simulink model "kalmanAndroidAHRS"  (R2019b)
settings: Solver=FixedStepAuto  StartTime=0.0  StopTime=40  RelTol=1e-3
InitFcn:
  | Ts=0.01
undefined symbols (not defined in the file): Accel, AHRS_Ang_Vel, AHRS_Attitude, Alt, AttiudeFiltered, fdesignblkfcn, gcbh, Gyro, Heading_Angle, kalman, kalman_clean, Mag, Pitch_Angle, Pitch_Rate, Roll_Angle, Roll_Rate, Slider, Static_Orientation, Yaw_Rate
libraries: androiduilib x15, simulink_extras x6, androidsensorlib x5, mspfiltlib x1, aerolibatmos2 x1
PreSaveFcn:
  | set_param(gcs, 'Location',[35 56 895 605])
settings Model: SimulationMode=external  ExtModeTrigDuration=100  Creator=The MathWorks, Inc.  LastModifiedBy=alireza
settings DataIOCC: LimitDataPoints=on  SaveFormat=Array  ReturnWorkspaceOutputs=off
settings OptimizationCC: LifeSpan=1  MaxStackSize=64
settings DebuggingCC: UnderspecifiedInitializationDetection=Classic  MergeDetectMultiDrivingBlocksExec=none  ParameterPrecisionLossMsg=none  AllowSymbolicDim=off  SFUnexpectedBacktrackingDiag=warning  SFNoUnconditionalDefaultTransitionDiag=warning  SFExecutionAtInitializationDiag=none  ArithmeticOperatorsInVariantConditions=warning
settings HardwareCC: ProdBitPerPointer=32  ProdBitPerSizeT=32  ProdBitPerPtrDiffT=32  ProdLargestAtomicInteger=Long  ProdLargestAtomicFloat=Double  ProdWordSize=32  ProdHWDeviceType=ARM Compatible->ARM Cortex  TargetLargestAtomicInteger=Long  TargetLargestAtomicFloat=Double  TargetEndianess=LittleEndian  TargetHWDeviceType=ARM Compatible->ARM Cortex
settings ModelReferenceCC: PropagateSignalLabelsOutOfModel=off
settings SFSimCC: SimUseLocalCustomCode=off  CustomCodeUndefinedFunction=UseInterfaceOnly
settings RTWCC: SystemTargetFile=ert.tlc  HardwareBoard=Android Device  TLCOptions="-aInlineSetEventsForThisBaseRateFcn=TLC_FALSE -aSuppressMultiTaskScheduler=TLC_FALSE  -aRateBasedStepFcn=0"  TemplateMakefile=ert_default_tmf  GenerateReport=on  RTWVerbose=off  RTWUseLocalCustomCode=off  Toolchain=Android SDK/NDK Tools  LaunchReport=on
settings CodeAppCC: ForceParamTrailComments=on  OperatorAnnotations=on  MangleLength=10  StateflowObjectComments=on  MATLABSourceComments=on
settings ERTTargetCC: MultiwordLength=2048  ERTCustomFileBanners=off  SupportContinuousTime=on  SupportNonInlinedSFcns=on  RemoveResetFunc=off  SupportVariableSizeSignals=on  ModelStepFunctionPrototypeControlCompliant=off
settings ConfigComp: CovMetricSettings=dw  CovHtmlReporting=on  CovSaveCumulativeToWorkspaceVar=on  CovSaveSingleToWorkspaceVar=on  CovExternalEMLEnable=off  CovSFcnEnable=off

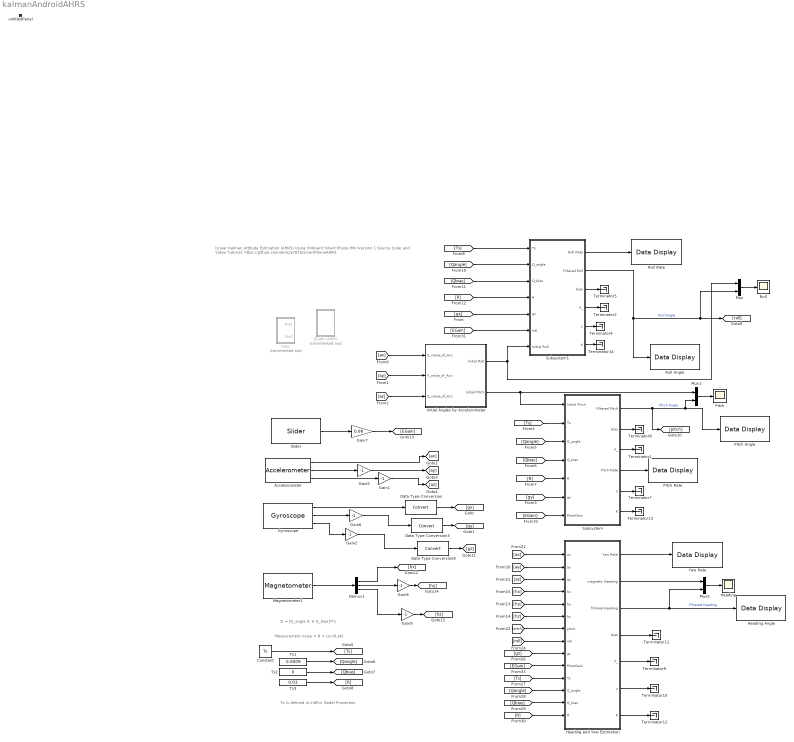
== system kalmanAndroidAHRS ==
  note: Ts is defined in initFcn Model Properties
  note: Linear Kalman Attitude Estimation (AHRS)
      | Using Onboard Smart Phone IMU Version 1
      | Source Code and Video Tutorial:
      | https://github.com/alireza787b/smartPhoneAHRS
  note: Measurement noise = R = cov(0,ek)
  note: Q = [Q_angle 0; 0 Q_bias]*Ts
  Accelerometer : androidsensorlib/Accelerometer  OutputVector=off  SampleTime=Ts  BlockPlatform=Android
      settings: SourceProductBaseCode=ANDROID
  BuiltIn AHRS : Subsystem  Commented=on
  Constant : Constant  Value=Ts
  Data Type Conversion : DataTypeConversion
  Data Type Conversion3 : DataTypeConversion
  Data Type Conversion8 : DataTypeConversion
  Demux1 : Demux  Outputs=3
  Gain{1..2,5..6,8..9} (6 alike) : Gain  Gain=-1
  Gain7 : Gain  Gain=0.98
  Gyroscope : androidsensorlib/Gyroscope  OutputVector=off  SampleTime=Ts  BlockPlatform=Android
      settings: SourceProductBaseCode=ANDROID
  Heading : Scope
  Heading Angle : androiduilib/Data Display  DataDisplayId=kalman_clean/Heading_Angle  Format=Float  Precision=6  SimulateUsing=Code generation  blockPlatform=Android
      settings: SourceProductBaseCode=ANDROID
  Heading and Yaw Estimation : Subsystem
  Initial Angles by Accelerometer : Subsystem
  Magnetometer1 : androidsensorlib/Magnetometer  SampleTime=0.01  SimulateUsing=Code generation
      settings: SourceProductBaseCode=ANDROID
  Mux : Mux  Inputs=2
  Mux1 : Mux  Inputs=2
  Mux5 : Mux  Inputs=2
  Pitch : Scope
  Pitch Angle : androiduilib/Data Display  DataDisplayId=kalman_clean/Pitch_Angle  Format=Float  Precision=6  SimulateUsing=Code generation  blockPlatform=Android
      settings: SourceProductBaseCode=ANDROID
  Pitch Rate : androiduilib/Data Display  DataDisplayId=kalman_clean/Pitch_Rate  Format=Float  Precision=6  SimulateUsing=Code generation  blockPlatform=Android
      settings: SourceProductBaseCode=ANDROID
  Roll : Scope
  Roll Angle : androiduilib/Data Display  DataDisplayId=kalman_clean/Roll_Angle  Format=Float  Precision=6  SimulateUsing=Code generation  blockPlatform=Android
      settings: SourceProductBaseCode=ANDROID
  Roll Rate : androiduilib/Data Display  DataDisplayId=kalman_clean/Roll_Rate  Format=Float  Precision=6  SimulateUsing=Code generation  blockPlatform=Android
      settings: SourceProductBaseCode=ANDROID
  Slider : androiduilib/Slider  Min=0  Value=1  Max=2  Resolution=0.1  SliderId=kalman_clean/Slider  SampleTime=0.1  BlockPlatform=Android
      settings: SourceProductBaseCode=ANDROID
  Subsystem : Subsystem
  Subsystem1 : Subsystem
  Terminator{1..2,4..5,7..14} (12 alike) : Terminator
  Ts1 : Constant  Value=0.0009
  Ts2 : Constant  Value=0
  Ts3 : Constant  Value=0.03
  Yaw Rate : androiduilib/Data Display  DataDisplayId=kalman_clean/Yaw_Rate  Format=Float  Precision=6  SimulateUsing=Code generation  blockPlatform=Android
      settings: SourceProductBaseCode=ANDROID
  misc : Subsystem  Commented=on
  untitledPanel : Subsystem  Tag=HiddenForWebPanel  IsWebBlockPanel=on
  wires:
  Accelerometer/3 -> Gain1/1
  Accelerometer/1 -> [ax]
  Accelerometer/2 -> Gain5/1
  Gyroscope/2 -> Gain6/1
  Gyroscope/3 -> Gain2/1
  Gyroscope/1 -> Data Type Conversion/1
  Data Type Conversion/1 -> [gx]
  Data Type Conversion3/1 -> [gy]
  Gain6/1 -> Data Type Conversion3/1
  Mux/1 -> Roll/1
  Mux1/1 -> Pitch/1
  Constant/1 -> [Ts]
  Ts2/1 -> [Qbias]
  Ts1/1 -> [Qangle]
  Ts3/1 -> [R]
  Magnetometer1/1 -> Demux1/1
  Data Type Conversion8/1 -> [gz]
  Mux5/1 -> Heading/1
  Slider/1 -> Gain7/1
  Gain5/1 -> [ay]
  Demux1/1 -> [hx]
  Demux1/2 -> Gain8/1
  Demux1/3 -> Gain9/1
  Gain8/1 -> [hy]
  Gain1/1 -> [az]
  Gain2/1 -> Data Type Conversion8/1
  Gain9/1 -> [hz]
  Gain7/1 -> [EGain]
  [ax] -> Heading and Yaw Estimation/1(ax)
  [ay] -> Heading and Yaw Estimation/2(ay)
  [az] -> Heading and Yaw Estimation/3(az)
  [hx] -> Heading and Yaw Estimation/4(hx)
  [hy] -> Heading and Yaw Estimation/5(hy)
  [hz] -> Heading and Yaw Estimation/6(hz)
  [pitch] -> Heading and Yaw Estimation/7(pitch)
  [roll] -> Heading and Yaw Estimation/8(roll)
  [gz] -> Heading and Yaw Estimation/9(gz)
  [EGain] -> Heading and Yaw Estimation/10(filterGain)
  [Ts] -> Heading and Yaw Estimation/11(Ts)
  [Qangle] -> Heading and Yaw Estimation/12(Q_angle)
  [Qbias] -> Heading and Yaw Estimation/13(Q_bias)
  [R] -> Heading and Yaw Estimation/14(R)
  Heading and Yaw Estimation/1(Yaw Rate) -> Yaw Rate/1
  Heading and Yaw Estimation/2(magnetic Heading) -> Mux5/1
  Heading and Yaw Estimation/4(bias) -> Terminator11/1
  Heading and Yaw Estimation/5(P_) -> Terminator9/1
  Heading and Yaw Estimation/6(y) -> Terminator10/1
  Heading and Yaw Estimation/7(K) -> Terminator12/1
  Heading and Yaw Estimation/3(filtered Heading) -> Mux5/2, Heading Angle/1  "Filtered Heading"
  Subsystem/1(Filtered Pitch) -> [pitch], Pitch Angle/1, Mux1/2  "Pitch Angle"
  [Ts] -> Subsystem/2(Ts)
  [Qangle] -> Subsystem/3(Q_angle)
  [Qbias] -> Subsystem/4(Q_bias)
  [R] -> Subsystem/5(R)
  [gy] -> Subsystem/6(gy)
  [EGain] -> Subsystem/7(filterGain)
  Subsystem/2(bias) -> Terminator8/1
  Subsystem/3(P_) -> Terminator1/1
  Subsystem/4(Pitch Rate) -> Pitch Rate/1
  Subsystem/5(y) -> Terminator7/1
  Subsystem/6(K) -> Terminator13/1
  Subsystem1/2(Filtered Roll) -> [roll], Mux/2, Roll Angle/1  "Roll Angle"
  Subsystem1/1(Roll Rate) -> Roll Rate/1
  [Ts] -> Subsystem1/1(Ts)
  [Qangle] -> Subsystem1/2(Q_angle)
  [Qbias] -> Subsystem1/3(Q_bias)
  [R] -> Subsystem1/4(R)
  [gx] -> Subsystem1/5(gx)
  [EGain] -> Subsystem1/6(In6)
  Subsystem1/3(bias) -> Terminator5/1
  Subsystem1/4(P_) -> Terminator2/1
  Subsystem1/5(y) -> Terminator4/1
  Subsystem1/6(K) -> Terminator14/1
  Initial Angles by Accelerometer/1(Initial Roll) -> Mux/1, Subsystem1/7(Initial Roll)
  Initial Angles by Accelerometer/2(Initial Pitch) -> Subsystem/1(Initial Pitch), Mux1/1
  [ax] -> Initial Angles by Accelerometer/1(X_value_of_Acc)
  [ay] -> Initial Angles by Accelerometer/2(Y_value_of_Acc)
  [az] -> Initial Angles by Accelerometer/3(Z_value_of_Acc)

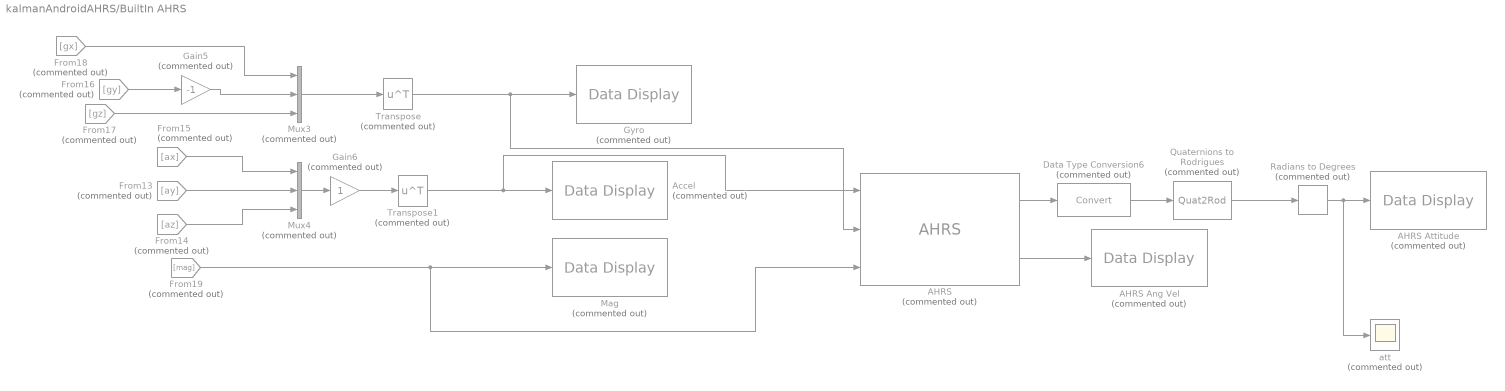
== system kalmanAndroidAHRS/BuiltIn AHRS ==
  AHRS : mspfiltlib/AHRS  Commented=on  DispRefFrame=NED  DecimationFactor=1  InitialProcessNoise=ahrsfilter.defaultProcessNoise  OrientationFormat=quaternion  SimulateUsing=Code generation  AccelerometerNoise=7.7792e-07  GyroscopeNoise=3.7046e-08  MagnetometerNoise=0.1  GyroscopeDriftNoise=3.0462e-13  LinearAccelerationNoise=0.0096236100000000012  MagneticDisturbanceNoise=0.5  LinearAccelerationDecayFactor=0.5  MagneticDisturbanceDecayFactor=0.5  ExpectedMagneticFieldStrength=50
      settings: SourceProductBaseCode=TF,NV
  AHRS Ang Vel : androiduilib/Data Display  Commented=on  DataDisplayId=kalman/AHRS_Ang_Vel  Format=Float  Precision=6  SimulateUsing=Code generation  blockPlatform=Android
      settings: SourceProductBaseCode=ANDROID
  AHRS Attitude : androiduilib/Data Display  Commented=on  DataDisplayId=kalman/AHRS_Attitude  Format=Float  Precision=6  SimulateUsing=Code generation  blockPlatform=Android
      settings: SourceProductBaseCode=ANDROID
  Accel : androiduilib/Data Display  Commented=on  DataDisplayId=kalman/Accel  Format=Float  Precision=6  SimulateUsing=Code generation  blockPlatform=Android
      settings: SourceProductBaseCode=ANDROID
  Data Type Conversion6 : DataTypeConversion  Commented=on
  From13 : From  Commented=on  GotoTag=ay
  From14 : From  Commented=on  GotoTag=az
  From15 : From  Commented=on  GotoTag=ax
  From16 : From  Commented=on  GotoTag=gy
  From17 : From  Commented=on  GotoTag=gz
  From18 : From  Commented=on  GotoTag=gx
  From19 : From  Commented=on  GotoTag=mag
  Gain5 : Gain  Commented=on  Gain=-1
  Gain6 : Gain  Commented=on
  Gyro : androiduilib/Data Display  Commented=on  DataDisplayId=kalman/Gyro  Format=Float  Precision=6  SimulateUsing=Code generation  blockPlatform=Android
      settings: SourceProductBaseCode=ANDROID
  Mag : androiduilib/Data Display  Commented=on  DataDisplayId=kalman/Mag  Format=Float  Precision=6  SimulateUsing=Code generation  blockPlatform=Android
      settings: SourceProductBaseCode=ANDROID
  Mux3 : Mux  Commented=on  Inputs=3
  Mux4 : Mux  Commented=on  Inputs=3
  Quaternions to Rodrigues : Quat2Rod  Commented=on
  Radians to Degrees : simulink_extras/Transformations/Radians to Degrees  Commented=on
  Transpose : Math  Commented=on  Operator=transpose  SaturateOnIntegerOverflow=on
  Transpose1 : Math  Commented=on  Operator=transpose  SaturateOnIntegerOverflow=on
  att : Scope  Commented=on
  wires:
  From18/1 -> Mux3/1
  From14/1 -> Mux4/3
  AHRS/2 -> AHRS Ang Vel/1
  Transpose/1 -> AHRS/2, Gyro/1
  From17/1 -> Mux3/3
  Mux4/1 -> Gain6/1
  Transpose1/1 -> AHRS/1, Accel/1
  From15/1 -> Mux4/1
  From19/1 -> AHRS/3, Mag/1
  From13/1 -> Mux4/2
  AHRS/1 -> Data Type Conversion6/1
  Data Type Conversion6/1 -> Quaternions to Rodrigues/1
  Quaternions to Rodrigues/1 -> Radians to Degrees/1
  Radians to Degrees/1 -> att/1, AHRS Attitude/1
  Gain6/1 -> Transpose1/1
  Gain5/1 -> Mux3/2
  From16/1 -> Gain5/1
  Mux3/1 -> Transpose/1

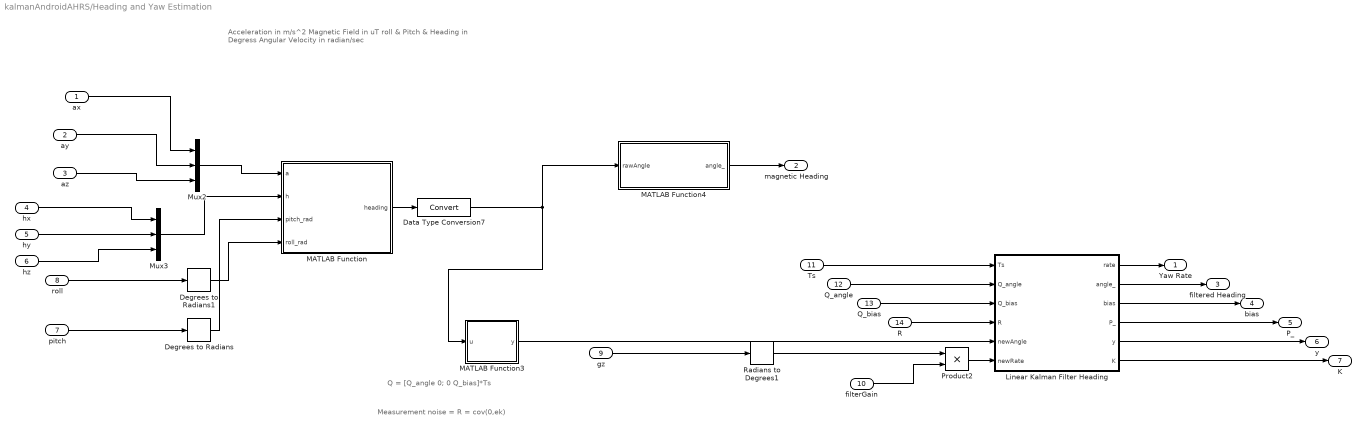
== system kalmanAndroidAHRS/Heading and Yaw Estimation ==
  note: Acceleration in m/s^2
      | Magnetic Field in uT
      | roll & Pitch & Heading in Degress
      | Angular Velocity in radian/sec
  note: Measurement noise = R = cov(0,ek)
  note: Q = [Q_angle 0; 0 Q_bias]*Ts
  ax : Inport
  ay : Inport  Port=2
  az : Inport  Port=3
  hx : Inport  Port=4
  hy : Inport  Port=5
  hz : Inport  Port=6
  pitch : Inport  Port=7
  roll : Inport  Port=8
  gz : Inport  Port=9
  filterGain : Inport  Port=10
  Ts : Inport  Port=11
  Q_angle : Inport  Port=12
  Q_bias : Inport  Port=13
  R : Inport  Port=14
  Data Type Conversion7 : DataTypeConversion
  Degrees to Radians : simulink_extras/Transformations/Degrees to Radians
  Degrees to Radians1 : simulink_extras/Transformations/Degrees to Radians
  Linear Kalman Filter Heading : MATLAB Function  TreatAsAtomicUnit=on
  MATLAB Function : MATLAB Function  TreatAsAtomicUnit=on
  MATLAB Function3 : MATLAB Function  TreatAsAtomicUnit=on
  MATLAB Function4 : MATLAB Function  TreatAsAtomicUnit=on
  Mux2 : Mux  Inputs=3
  Mux3 : Mux  Inputs=3
  Product2 : Product
  Radians to Degrees1 : simulink_extras/Transformations/Radians to Degrees
  Yaw Rate : Outport
  magnetic Heading : Outport  Port=2
  filtered Heading : Outport  Port=3
  bias : Outport  Port=4
  P_ : Outport  Port=5
  y : Outport  Port=6
  K : Outport  Port=7
  wires:
  MATLAB Function3/1(y) -> Linear Kalman Filter Heading/5(newAngle)
  Mux2/1 -> MATLAB Function/1(a)
  hy/1 -> Mux3/2
  Degrees to Radians/1 -> MATLAB Function/3(pitch_rad)
  Data Type Conversion7/1 -> MATLAB Function3/1(u), MATLAB Function4/1(rawAngle)
  Linear Kalman Filter Heading/2(angle_) -> filtered Heading/1
  Product2/1 -> Linear Kalman Filter Heading/6(newRate)
  Linear Kalman Filter Heading/6(K) -> K/1
  MATLAB Function/1(heading) -> Data Type Conversion7/1
  Radians to Degrees1/1 -> Product2/1
  Degrees to Radians1/1 -> MATLAB Function/4(roll_rad)
  Mux3/1 -> MATLAB Function/2(h)
  MATLAB Function4/1(angle_) -> magnetic Heading/1
  ay/1 -> Mux2/2
  ax/1 -> Mux2/1
  Q_angle/1 -> Linear Kalman Filter Heading/2(Q_angle)
  gz/1 -> Radians to Degrees1/1
  Ts/1 -> Linear Kalman Filter Heading/1(Ts)
  az/1 -> Mux2/3
  R/1 -> Linear Kalman Filter Heading/4(R)
  Linear Kalman Filter Heading/3(bias) -> bias/1
  Linear Kalman Filter Heading/1(rate) -> Yaw Rate/1
  hz/1 -> Mux3/3
  hx/1 -> Mux3/1
  filterGain/1 -> Product2/2
  Q_bias/1 -> Linear Kalman Filter Heading/3(Q_bias)
  roll/1 -> Degrees to Radians1/1
  pitch/1 -> Degrees to Radians/1
  Linear Kalman Filter Heading/5(y) -> y/1
  Linear Kalman Filter Heading/4(P_) -> P_/1

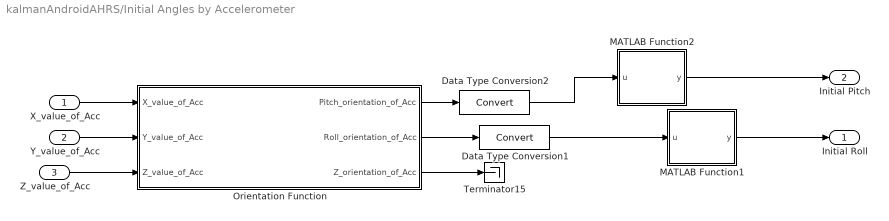
== system kalmanAndroidAHRS/Initial Angles by Accelerometer ==
  X_value_of_Acc : Inport
  Y_value_of_Acc : Inport  Port=2
  Z_value_of_Acc : Inport  Port=3
  Data Type Conversion1 : DataTypeConversion
  Data Type Conversion2 : DataTypeConversion
  MATLAB Function1 : MATLAB Function  TreatAsAtomicUnit=on
  MATLAB Function2 : MATLAB Function  TreatAsAtomicUnit=on
  Orientation Function : MATLAB Function  TreatAsAtomicUnit=on
  Terminator15 : Terminator
  Initial Roll : Outport
  Initial Pitch : Outport  Port=2
  wires:
  Orientation Function/2(Roll_orientation_of_Acc) -> Data Type Conversion1/1
  Data Type Conversion1/1 -> MATLAB Function1/1(u)
  X_value_of_Acc/1 -> Orientation Function/1(X_value_of_Acc)
  Y_value_of_Acc/1 -> Orientation Function/2(Y_value_of_Acc)
  Orientation Function/1(Pitch_orientation_of_Acc) -> Data Type Conversion2/1
  MATLAB Function2/1(y) -> Initial Pitch/1
  Data Type Conversion2/1 -> MATLAB Function2/1(u)
  Orientation Function/3(Z_orientation_of_Acc) -> Terminator15/1
  Z_value_of_Acc/1 -> Orientation Function/3(Z_value_of_Acc)
  MATLAB Function1/1(y) -> Initial Roll/1

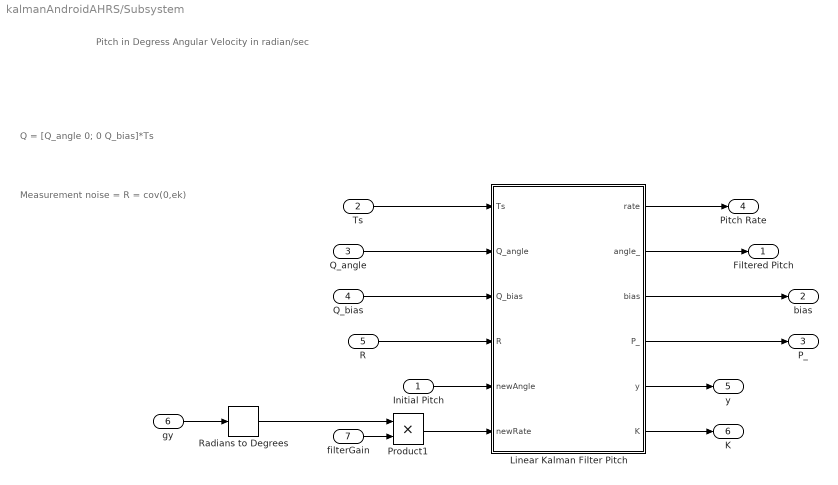
== system kalmanAndroidAHRS/Subsystem ==
  note: Pitch in Degress
      | Angular Velocity in radian/sec
  note: Measurement noise = R = cov(0,ek)
  note: Q = [Q_angle 0; 0 Q_bias]*Ts
  Initial Pitch : Inport
  Ts : Inport  Port=2
  Q_angle : Inport  Port=3
  Q_bias : Inport  Port=4
  R : Inport  Port=5
  gy : Inport  Port=6
  filterGain : Inport  Port=7
  Linear Kalman Filter Pitch : MATLAB Function  TreatAsAtomicUnit=on
  Product1 : Product
  Radians to Degrees : simulink_extras/Transformations/Radians to Degrees
  Filtered Pitch : Outport
  bias : Outport  Port=2
  P_ : Outport  Port=3
  Pitch Rate : Outport  Port=4
  y : Outport  Port=5
  K : Outport  Port=6
  wires:
  Linear Kalman Filter Pitch/3(bias) -> bias/1
  Linear Kalman Filter Pitch/1(rate) -> Pitch Rate/1
  Product1/1 -> Linear Kalman Filter Pitch/6(newRate)
  Radians to Degrees/1 -> Product1/1
  filterGain/1 -> Product1/2
  gy/1 -> Radians to Degrees/1
  Linear Kalman Filter Pitch/5(y) -> y/1
  Linear Kalman Filter Pitch/4(P_) -> P_/1
  Ts/1 -> Linear Kalman Filter Pitch/1(Ts)
  Q_bias/1 -> Linear Kalman Filter Pitch/3(Q_bias)
  Q_angle/1 -> Linear Kalman Filter Pitch/2(Q_angle)
  Linear Kalman Filter Pitch/2(angle_) -> Filtered Pitch/1
  Linear Kalman Filter Pitch/6(K) -> K/1
  R/1 -> Linear Kalman Filter Pitch/4(R)
  Initial Pitch/1 -> Linear Kalman Filter Pitch/5(newAngle)

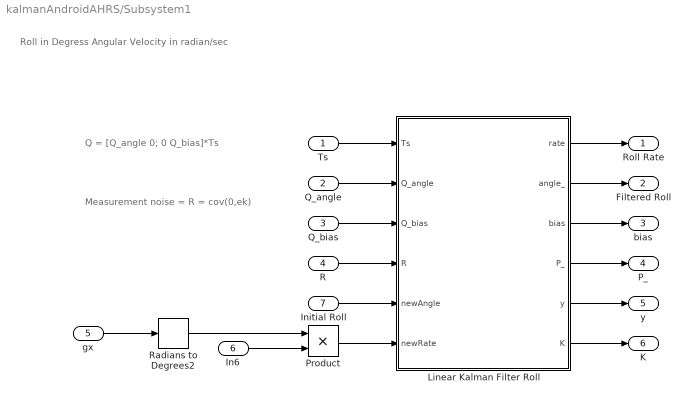
== system kalmanAndroidAHRS/Subsystem1 ==
  note: Measurement noise = R = cov(0,ek)
  note: Q = [Q_angle 0; 0 Q_bias]*Ts
  note: Roll in Degress
      | Angular Velocity in radian/sec
  Ts : Inport
  Q_angle : Inport  Port=2
  Q_bias : Inport  Port=3
  R : Inport  Port=4
  gx : Inport  Port=5
  In6 : Inport  Port=6
  Initial Roll : Inport  Port=7
  Linear Kalman Filter Roll : MATLAB Function  TreatAsAtomicUnit=on
  Product : Product
  Radians to Degrees2 : simulink_extras/Transformations/Radians to Degrees
  Roll Rate : Outport
  Filtered Roll : Outport  Port=2
  bias : Outport  Port=3
  P_ : Outport  Port=4
  y : Outport  Port=5
  K : Outport  Port=6
  wires:
  Linear Kalman Filter Roll/4(P_) -> P_/1
  Linear Kalman Filter Roll/1(rate) -> Roll Rate/1
  In6/1 -> Product/2
  Radians to Degrees2/1 -> Product/1
  Linear Kalman Filter Roll/3(bias) -> bias/1
  Linear Kalman Filter Roll/5(y) -> y/1
  Product/1 -> Linear Kalman Filter Roll/6(newRate)
  Initial Roll/1 -> Linear Kalman Filter Roll/5(newAngle)
  Ts/1 -> Linear Kalman Filter Roll/1(Ts)
  Linear Kalman Filter Roll/2(angle_) -> Filtered Roll/1
  R/1 -> Linear Kalman Filter Roll/4(R)
  Q_bias/1 -> Linear Kalman Filter Roll/3(Q_bias)
  Q_angle/1 -> Linear Kalman Filter Roll/2(Q_angle)
  Linear Kalman Filter Roll/6(K) -> K/1
  gx/1 -> Radians to Degrees2/1

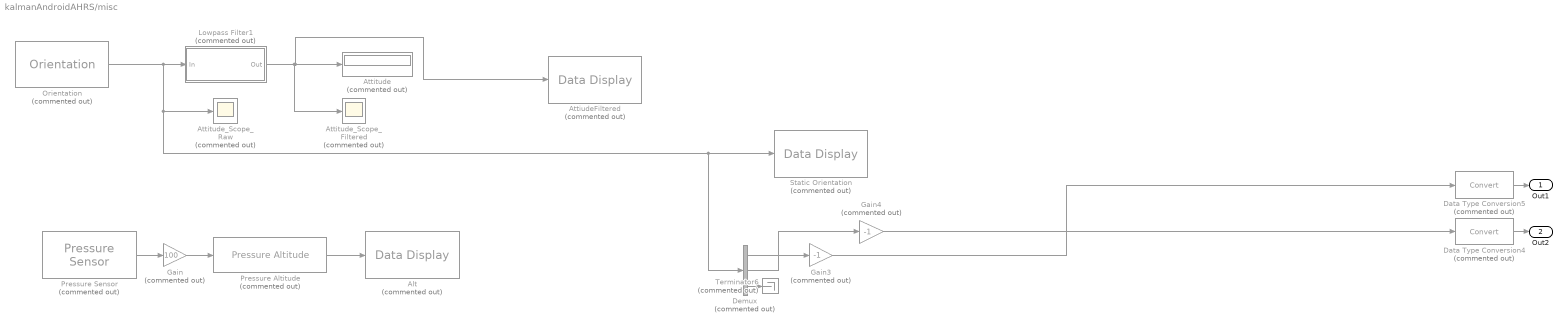
== system kalmanAndroidAHRS/misc ==
  Alt : androiduilib/Data Display  Commented=on  DataDisplayId=kalman/Alt  Format=Float  Precision=6  SimulateUsing=Code generation  blockPlatform=Android
      settings: SourceProductBaseCode=ANDROID
  Attitude : Display  Commented=on
  Attitude_Scope_Filtered : Scope  Commented=on
  Attitude_Scope_Raw : Scope  Commented=on
  AttiudeFiltered : androiduilib/Data Display  Commented=on  DataDisplayId=kalman/AttiudeFiltered  Format=Float  Precision=6  SimulateUsing=Code generation  blockPlatform=Android
      settings: SourceProductBaseCode=ANDROID
  Data Type Conversion4 : DataTypeConversion  Commented=on
  Data Type Conversion5 : DataTypeConversion  Commented=on
  Demux : Demux  Commented=on  Outputs=3
  Gain : Gain  Commented=on  Gain=100
  Gain3 : Gain  Commented=on  Gain=-1
  Gain4 : Gain  Commented=on  Gain=-1
  Lowpass Filter1 : Subsystem  Commented=on  DialogController=fdesignblkfcn  InitFcn=fdesignblkfcn(gcbh, {'InitFcn'});  mask(Lowpass Filter){}
      mask help: Design a lowpass filter
      settings: CopyFcn=fdesignblkfcn(gcbh, {'CopyFcn'});
      mask Help: helpview(mapfilelocation('dsp'), 'dsplowpassfilter');
      mask Display: disp('Lowpass')
  Orientation : androidsensorlib/Orientation  Commented=on  SampleTime=Ts  SimulateUsing=Code generation
      settings: SourceProductBaseCode=ANDROID
  Pressure Altitude : aerolibatmos2/Pressure Altitude  Commented=on  units=Metric (MKS)  action=Warning
      settings: SourceProductBaseCode=AE
  Pressure Sensor : androidsensorlib/Pressure Sensor  Commented=on  SampleTime=1  BlockPlatform=Android
      settings: SourceProductBaseCode=ANDROID
  Static Orientation : androiduilib/Data Display  Commented=on  DataDisplayId=kalman/Static_Orientation  Format=Float  Precision=6  SimulateUsing=Code generation  blockPlatform=Android
      settings: SourceProductBaseCode=ANDROID
  Terminator6 : Terminator  Commented=on
  Out1 : Outport
  Out2 : Outport  Port=2
  wires:
  Data Type Conversion4/1 -> Out2/1
  Lowpass Filter1/1(Out) -> Attitude_Scope_Filtered/1, AttiudeFiltered/1, Attitude/1
  Gain/1 -> Pressure Altitude/1
  Pressure Sensor/1 -> Gain/1
  Demux/2 -> Gain4/1
  Gain3/1 -> Data Type Conversion5/1
  Orientation/1 -> Attitude_Scope_Raw/1, Demux/1, Static Orientation/1, Lowpass Filter1/1(In)
  Data Type Conversion5/1 -> Out1/1
  Demux/1 -> Gain3/1
  Pressure Altitude/1 -> Alt/1
  Demux/3 -> Terminator6/1
  Gain4/1 -> Data Type Conversion4/1

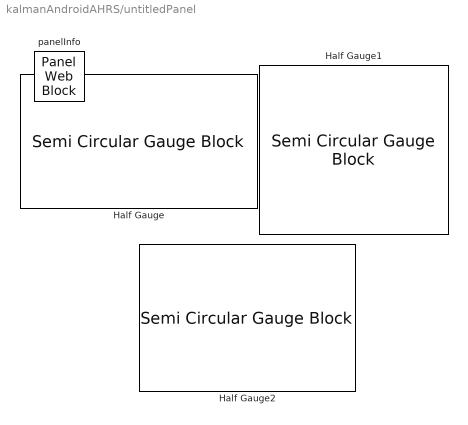
== system kalmanAndroidAHRS/untitledPanel ==
  Half Gauge : SemiCircularGaugeBlock  Tag=HiddenForWebPanel  PanelInfo="{\"panelId\":\"panelId-765474a9-9c5b-495a-8d41-f66c7c8f1f34\",\"type\":\"panelChild\",\"version\":\"2019b\",\"zIndex\":1500004}"  ScaleMin=-90  ScaleMax=+90
  Half Gauge1 : SemiCircularGaugeBlock  Tag=HiddenForWebPanel  PanelInfo="{\"panelId\":\"panelId-765474a9-9c5b-495a-8d41-f66c7c8f1f34\",\"type\":\"panelChild\",\"version\":\"2019b\",\"zIndex\":1500001}"  ScaleMin=-90  ScaleMax=+90
  Half Gauge2 : SemiCircularGaugeBlock  Tag=HiddenForWebPanel  PanelInfo="{\"panelId\":\"panelId-765474a9-9c5b-495a-8d41-f66c7c8f1f34\",\"type\":\"panelChild\",\"version\":\"2019b\",\"zIndex\":1500002}"  ScaleMax=360
  panelInfo : PanelWebBlock  Tag=HiddenForWebPanel  PanelInfo="{\"compacted\":true,\"height\":441,\"labels\":{\"label8769572146\":{\"left\":\"231\",\"settings\":{\"backgroundColor\":\"rgba(0, 0, 0, 0)\",\"bold\":false,\"font\":\"Arial\",\"fontColor\":\"black\",\"fontSize\":1.48,\"italicized\":false,\"underlined\":false},\"text\":\"\\u001B\\u001B\",\"top\":\"319\"}},\"left\":1290,\"panelId\":\"panelId-765474a9-9c5b-495a-8d41-f66c7c8f1f34\",\"top\":463,\"type\":\"panel\",\"version\":\"2019b\",\"visible\":true,\"width\":432,\"zIndex\":1500001}"  PanelSnapshot=<binary blob, 68872 chars, not shown>

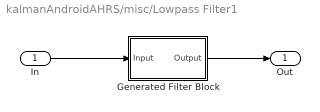
== system kalmanAndroidAHRS/misc/Lowpass Filter1 ==
  In : Inport
  Generated Filter Block : Subsystem  Tag=FilterWizardSubSystem
      settings: ErrorFcn=dspFilterRealizedInBasicElemsAlgLoopErrFcnCallback
  Out : Outport
  wires:
  In/1 -> Generated Filter Block/1(Input)
  Generated Filter Block/1(Output) -> Out/1

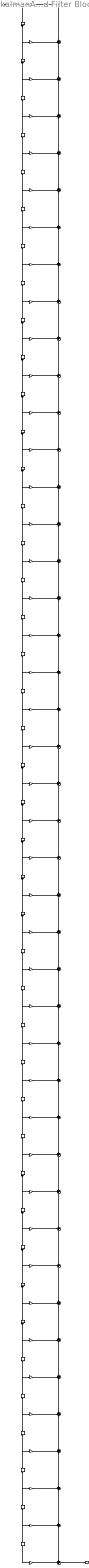
== system kalmanAndroidAHRS/misc/Lowpass Filter1/Generated Filter Block ==
  Input : Inport
  BodyDelay{2..43} (42 alike) : Delay  DelayLength=1  InitialCondition=0
  BodyLSum{2..43} (42 alike) : Sum  Inputs=++|  RndMeth=Nearest  SaturateOnIntegerOverflow=on  OutDataTypeStr=Inherit: Same as first input
  b(1) : Gain  Gain=-0.00242287385232693503  ParamDataTypeStr=double  RndMeth=Nearest  SaturateOnIntegerOverflow=on  OutDataTypeStr=Inherit: Same as input
  b(10) : Gain  Gain=-0.0101212347032790025  ParamDataTypeStr=double  RndMeth=Nearest  SaturateOnIntegerOverflow=on  OutDataTypeStr=Inherit: Same as input
  b(11) : Gain  Gain=-0.0182735187337824609  ParamDataTypeStr=double  RndMeth=Nearest  SaturateOnIntegerOverflow=on  OutDataTypeStr=Inherit: Same as input
  b(12) : Gain  Gain=0.0114319620717779676  ParamDataTypeStr=double  RndMeth=Nearest  SaturateOnIntegerOverflow=on  OutDataTypeStr=Inherit: Same as input
  b(13) : Gain  Gain=0.026175888580407581  ParamDataTypeStr=double  RndMeth=Nearest  SaturateOnIntegerOverflow=on  OutDataTypeStr=Inherit: Same as input
  b(14) : Gain  Gain=-0.0124890278353230171  ParamDataTypeStr=double  RndMeth=Nearest  SaturateOnIntegerOverflow=on  OutDataTypeStr=Inherit: Same as input
  b(15) : Gain  Gain=-0.0379966231454636413  ParamDataTypeStr=double  RndMeth=Nearest  SaturateOnIntegerOverflow=on  OutDataTypeStr=Inherit: Same as input
  b(16) : Gain  Gain=0.0133889451993669008  ParamDataTypeStr=double  RndMeth=Nearest  SaturateOnIntegerOverflow=on  OutDataTypeStr=Inherit: Same as input
  b(17) : Gain  Gain=0.0581554658147298703  ParamDataTypeStr=double  RndMeth=Nearest  SaturateOnIntegerOverflow=on  OutDataTypeStr=Inherit: Same as input
  b(18) : Gain  Gain=-0.0140480435158088935  ParamDataTypeStr=double  RndMeth=Nearest  SaturateOnIntegerOverflow=on  OutDataTypeStr=Inherit: Same as input
  b(19) : Gain  Gain=-0.102724668578821676  ParamDataTypeStr=double  RndMeth=Nearest  SaturateOnIntegerOverflow=on  OutDataTypeStr=Inherit: Same as input
  b(2) : Gain  Gain=-0.00208324498207925878  ParamDataTypeStr=double  RndMeth=Nearest  SaturateOnIntegerOverflow=on  OutDataTypeStr=Inherit: Same as input
  b(20) : Gain  Gain=0.0144622757712384552  ParamDataTypeStr=double  RndMeth=Nearest  SaturateOnIntegerOverflow=on  OutDataTypeStr=Inherit: Same as input
  b(21) : Gain  Gain=0.317166497217694909  ParamDataTypeStr=double  RndMeth=Nearest  SaturateOnIntegerOverflow=on  OutDataTypeStr=Inherit: Same as input
  b(22) : Gain  Gain=0.485387646787325211  ParamDataTypeStr=double  RndMeth=Nearest  SaturateOnIntegerOverflow=on  OutDataTypeStr=Inherit: Same as input
  b(23) : Gain  Gain=0.317166497217694909  ParamDataTypeStr=double  RndMeth=Nearest  SaturateOnIntegerOverflow=on  OutDataTypeStr=Inherit: Same as input
  b(24) : Gain  Gain=0.0144622757712384552  ParamDataTypeStr=double  RndMeth=Nearest  SaturateOnIntegerOverflow=on  OutDataTypeStr=Inherit: Same as input
  b(25) : Gain  Gain=-0.102724668578821676  ParamDataTypeStr=double  RndMeth=Nearest  SaturateOnIntegerOverflow=on  OutDataTypeStr=Inherit: Same as input
  b(26) : Gain  Gain=-0.0140480435158088935  ParamDataTypeStr=double  RndMeth=Nearest  SaturateOnIntegerOverflow=on  OutDataTypeStr=Inherit: Same as input
  b(27) : Gain  Gain=0.0581554658147298703  ParamDataTypeStr=double  RndMeth=Nearest  SaturateOnIntegerOverflow=on  OutDataTypeStr=Inherit: Same as input
  b(28) : Gain  Gain=0.0133889451993669008  ParamDataTypeStr=double  RndMeth=Nearest  SaturateOnIntegerOverflow=on  OutDataTypeStr=Inherit: Same as input
  b(29) : Gain  Gain=-0.0379966231454636413  ParamDataTypeStr=double  RndMeth=Nearest  SaturateOnIntegerOverflow=on  OutDataTypeStr=Inherit: Same as input
  b(3) : Gain  Gain=0.00677034464011870129  ParamDataTypeStr=double  RndMeth=Nearest  SaturateOnIntegerOverflow=on  OutDataTypeStr=Inherit: Same as input
  b(30) : Gain  Gain=-0.0124890278353230171  ParamDataTypeStr=double  RndMeth=Nearest  SaturateOnIntegerOverflow=on  OutDataTypeStr=Inherit: Same as input
  b(31) : Gain  Gain=0.026175888580407581  ParamDataTypeStr=double  RndMeth=Nearest  SaturateOnIntegerOverflow=on  OutDataTypeStr=Inherit: Same as input
  b(32) : Gain  Gain=0.0114319620717779676  ParamDataTypeStr=double  RndMeth=Nearest  SaturateOnIntegerOverflow=on  OutDataTypeStr=Inherit: Same as input
  b(33) : Gain  Gain=-0.0182735187337824609  ParamDataTypeStr=double  RndMeth=Nearest  SaturateOnIntegerOverflow=on  OutDataTypeStr=Inherit: Same as input
  b(34) : Gain  Gain=-0.0101212347032790025  ParamDataTypeStr=double  RndMeth=Nearest  SaturateOnIntegerOverflow=on  OutDataTypeStr=Inherit: Same as input
  b(35) : Gain  Gain=0.0129828838088557105  ParamDataTypeStr=double  RndMeth=Nearest  SaturateOnIntegerOverflow=on  OutDataTypeStr=Inherit: Same as input
  b(36) : Gain  Gain=0.00925679761513798632  ParamDataTypeStr=double  RndMeth=Nearest  SaturateOnIntegerOverflow=on  OutDataTypeStr=Inherit: Same as input
  b(37) : Gain  Gain=-0.00840161718602687457  ParamDataTypeStr=double  RndMeth=Nearest  SaturateOnIntegerOverflow=on  OutDataTypeStr=Inherit: Same as input
  b(38) : Gain  Gain=-0.00623114541414451859  ParamDataTypeStr=double  RndMeth=Nearest  SaturateOnIntegerOverflow=on  OutDataTypeStr=Inherit: Same as input
  b(39) : Gain  Gain=0.0111170760810775926  ParamDataTypeStr=double  RndMeth=Nearest  SaturateOnIntegerOverflow=on  OutDataTypeStr=Inherit: Same as input
  b(4) : Gain  Gain=0.016731945423489044  ParamDataTypeStr=double  RndMeth=Nearest  SaturateOnIntegerOverflow=on  OutDataTypeStr=Inherit: Same as input
  b(40) : Gain  Gain=0.016731945423489044  ParamDataTypeStr=double  RndMeth=Nearest  SaturateOnIntegerOverflow=on  OutDataTypeStr=Inherit: Same as input
  b(41) : Gain  Gain=0.00677034464011870129  ParamDataTypeStr=double  RndMeth=Nearest  SaturateOnIntegerOverflow=on  OutDataTypeStr=Inherit: Same as input
  b(42) : Gain  Gain=-0.00208324498207925878  ParamDataTypeStr=double  RndMeth=Nearest  SaturateOnIntegerOverflow=on  OutDataTypeStr=Inherit: Same as input
  b(43) : Gain  Gain=-0.00242287385232693503  ParamDataTypeStr=double  RndMeth=Nearest  SaturateOnIntegerOverflow=on  OutDataTypeStr=Inherit: Same as input
  b(5) : Gain  Gain=0.0111170760810775926  ParamDataTypeStr=double  RndMeth=Nearest  SaturateOnIntegerOverflow=on  OutDataTypeStr=Inherit: Same as input
  b(6) : Gain  Gain=-0.00623114541414451859  ParamDataTypeStr=double  RndMeth=Nearest  SaturateOnIntegerOverflow=on  OutDataTypeStr=Inherit: Same as input
  b(7) : Gain  Gain=-0.00840161718602687457  ParamDataTypeStr=double  RndMeth=Nearest  SaturateOnIntegerOverflow=on  OutDataTypeStr=Inherit: Same as input
  b(8) : Gain  Gain=0.00925679761513798632  ParamDataTypeStr=double  RndMeth=Nearest  SaturateOnIntegerOverflow=on  OutDataTypeStr=Inherit: Same as input
  b(9) : Gain  Gain=0.0129828838088557105  ParamDataTypeStr=double  RndMeth=Nearest  SaturateOnIntegerOverflow=on  OutDataTypeStr=Inherit: Same as input
  Output : Outport
  wires:
  Input/1 -> b(1)/1, BodyDelay2/1
  b(1)/1 -> BodyLSum2/2
  BodyDelay2/1 -> b(2)/1, BodyDelay3/1
  b(2)/1 -> BodyLSum2/1
  BodyLSum2/1 -> BodyLSum3/2
  BodyDelay3/1 -> b(3)/1, BodyDelay4/1
  b(3)/1 -> BodyLSum3/1
  BodyLSum3/1 -> BodyLSum4/2
  BodyDelay4/1 -> b(4)/1, BodyDelay5/1
  b(4)/1 -> BodyLSum4/1
  BodyLSum4/1 -> BodyLSum5/2
  BodyDelay5/1 -> b(5)/1, BodyDelay6/1
  b(5)/1 -> BodyLSum5/1
  BodyLSum5/1 -> BodyLSum6/2
  BodyDelay6/1 -> b(6)/1, BodyDelay7/1
  b(6)/1 -> BodyLSum6/1
  BodyLSum6/1 -> BodyLSum7/2
  BodyDelay7/1 -> b(7)/1, BodyDelay8/1
  b(7)/1 -> BodyLSum7/1
  BodyLSum7/1 -> BodyLSum8/2
  BodyDelay8/1 -> b(8)/1, BodyDelay9/1
  b(8)/1 -> BodyLSum8/1
  BodyLSum8/1 -> BodyLSum9/2
  BodyDelay9/1 -> b(9)/1, BodyDelay10/1
  b(9)/1 -> BodyLSum9/1
  BodyLSum9/1 -> BodyLSum10/2
  BodyDelay10/1 -> b(10)/1, BodyDelay11/1
  b(10)/1 -> BodyLSum10/1
  BodyLSum10/1 -> BodyLSum11/2
  BodyDelay11/1 -> b(11)/1, BodyDelay12/1
  b(11)/1 -> BodyLSum11/1
  BodyLSum11/1 -> BodyLSum12/2
  BodyDelay12/1 -> b(12)/1, BodyDelay13/1
  b(12)/1 -> BodyLSum12/1
  BodyLSum12/1 -> BodyLSum13/2
  BodyDelay13/1 -> b(13)/1, BodyDelay14/1
  b(13)/1 -> BodyLSum13/1
  BodyLSum13/1 -> BodyLSum14/2
  BodyDelay14/1 -> b(14)/1, BodyDelay15/1
  b(14)/1 -> BodyLSum14/1
  BodyLSum14/1 -> BodyLSum15/2
  BodyDelay15/1 -> b(15)/1, BodyDelay16/1
  b(15)/1 -> BodyLSum15/1
  BodyLSum15/1 -> BodyLSum16/2
  BodyDelay16/1 -> b(16)/1, BodyDelay17/1
  b(16)/1 -> BodyLSum16/1
  BodyLSum16/1 -> BodyLSum17/2
  BodyDelay17/1 -> b(17)/1, BodyDelay18/1
  b(17)/1 -> BodyLSum17/1
  BodyLSum17/1 -> BodyLSum18/2
  BodyDelay18/1 -> b(18)/1, BodyDelay19/1
  b(18)/1 -> BodyLSum18/1
  BodyLSum18/1 -> BodyLSum19/2
  BodyDelay19/1 -> b(19)/1, BodyDelay20/1
  b(19)/1 -> BodyLSum19/1
  BodyLSum19/1 -> BodyLSum20/2
  BodyDelay20/1 -> b(20)/1, BodyDelay21/1
  b(20)/1 -> BodyLSum20/1
  BodyLSum20/1 -> BodyLSum21/2
  BodyDelay21/1 -> b(21)/1, BodyDelay22/1
  b(21)/1 -> BodyLSum21/1
  BodyLSum21/1 -> BodyLSum22/2
  BodyDelay22/1 -> b(22)/1, BodyDelay23/1
  b(22)/1 -> BodyLSum22/1
  BodyLSum22/1 -> BodyLSum23/2
  BodyDelay23/1 -> b(23)/1, BodyDelay24/1
  b(23)/1 -> BodyLSum23/1
  BodyLSum23/1 -> BodyLSum24/2
  BodyDelay24/1 -> b(24)/1, BodyDelay25/1
  b(24)/1 -> BodyLSum24/1
  BodyLSum24/1 -> BodyLSum25/2
  BodyDelay25/1 -> b(25)/1, BodyDelay26/1
  b(25)/1 -> BodyLSum25/1
  BodyLSum25/1 -> BodyLSum26/2
  BodyDelay26/1 -> b(26)/1, BodyDelay27/1
  b(26)/1 -> BodyLSum26/1
  BodyLSum26/1 -> BodyLSum27/2
  BodyDelay27/1 -> b(27)/1, BodyDelay28/1
  b(27)/1 -> BodyLSum27/1
  BodyLSum27/1 -> BodyLSum28/2
  BodyDelay28/1 -> b(28)/1, BodyDelay29/1
  b(28)/1 -> BodyLSum28/1
  BodyLSum28/1 -> BodyLSum29/2
  BodyDelay29/1 -> b(29)/1, BodyDelay30/1
  b(29)/1 -> BodyLSum29/1
  BodyLSum29/1 -> BodyLSum30/2
  BodyDelay30/1 -> b(30)/1, BodyDelay31/1
  b(30)/1 -> BodyLSum30/1
  BodyLSum30/1 -> BodyLSum31/2
  BodyDelay31/1 -> b(31)/1, BodyDelay32/1
  b(31)/1 -> BodyLSum31/1
  BodyLSum31/1 -> BodyLSum32/2
  BodyDelay32/1 -> b(32)/1, BodyDelay33/1
  b(32)/1 -> BodyLSum32/1
  BodyLSum32/1 -> BodyLSum33/2
  BodyDelay33/1 -> b(33)/1, BodyDelay34/1
  b(33)/1 -> BodyLSum33/1
  BodyLSum33/1 -> BodyLSum34/2
  BodyDelay34/1 -> b(34)/1, BodyDelay35/1
  b(34)/1 -> BodyLSum34/1
  BodyLSum34/1 -> BodyLSum35/2
  BodyDelay35/1 -> b(35)/1, BodyDelay36/1
  b(35)/1 -> BodyLSum35/1
  BodyLSum35/1 -> BodyLSum36/2
  BodyDelay36/1 -> b(36)/1, BodyDelay37/1
  b(36)/1 -> BodyLSum36/1
  BodyLSum36/1 -> BodyLSum37/2
  BodyDelay37/1 -> b(37)/1, BodyDelay38/1
  b(37)/1 -> BodyLSum37/1
  BodyLSum37/1 -> BodyLSum38/2
  BodyDelay38/1 -> b(38)/1, BodyDelay39/1
  b(38)/1 -> BodyLSum38/1
  BodyLSum38/1 -> BodyLSum39/2
  BodyDelay39/1 -> b(39)/1, BodyDelay40/1
  b(39)/1 -> BodyLSum39/1
  BodyLSum39/1 -> BodyLSum40/2
  BodyDelay40/1 -> b(40)/1, BodyDelay41/1
  b(40)/1 -> BodyLSum40/1
  BodyLSum40/1 -> BodyLSum41/2
  BodyDelay41/1 -> b(41)/1, BodyDelay42/1
  b(41)/1 -> BodyLSum41/1
  BodyLSum41/1 -> BodyLSum42/2
  BodyDelay42/1 -> b(42)/1, BodyDelay43/1
  b(42)/1 -> BodyLSum42/1
  BodyLSum42/1 -> BodyLSum43/1
  BodyDelay43/1 -> b(43)/1
  b(43)/1 -> BodyLSum43/2
  BodyLSum43/1 -> Output/1

== matlab function kalmanAndroidAHRS/Subsystem/Linear Kalman Filter Pitch ==
  data: Ts input; Q_angle input; Q_bias input; R input; newAngle input; rate output; newRate input; angle_ output; bias output; P_ output; y output; K output
% Algorithm -- implimentation of Linear-Kalman filter for a 6-DOF IMU using
% a single axis for testing. A single axis consisting of both anaccelerometer
% input and gyroscope input from IMU.
% Author: RM van Rensburg
% for IMU testing purposes
% Date: 26-04-2015
% Version: 1.0,tested on Matlab R2015a

function [rate,angle_,bias,P_,y,K] = Kalmanf(Ts,...
                                             Q_angle,Q_bias,R,...
                                             newAngle,...
                                             newRate)
                      
% Process noise covariance matrix  
Q = [Q_angle 0;0 Q_bias]*Ts;
A = [1  -Ts;0  1];
C = [1 0];
bias = 0.0;

rate = newRate - bias;

persistent angle;
if isempty(angle);angle = 0;
else angle = angle + (Ts * rate); 
end
angle_= angle;
                    
persistent P;
if isempty(P);P = [0 0 ; 0 0]; 
else P = A*P*A' + Q;
end
P_=P;

S = C*P*C' + R; % Estimate error 
K = (P_*C')/S; % Kalman gain
y = newAngle - angle_; % Angle difference 
xk = angle_ + K*y;
angle_ = xk(1); % - is added by me
bias = xk(2);
angle = angle_;

% Update the error covariance 
I = [1 0;0 1];
P_ = (I - K*C)*P_;
% or
% Joseph form (more stable)
% P_ = (I - K*C)*P_*(I - K*C) + K*R*K';
P = P_;

return

end

== matlab function kalmanAndroidAHRS/Initial Angles by Accelerometer/MATLAB Function2 ==
  data: u input; y output
function y = fcn(u)

if(isnan(u))
y=0;
else
y=u;
end

== matlab function kalmanAndroidAHRS/Initial Angles by Accelerometer/Orientation Function ==
  data: X_value_of_Acc input; Pitch_orientation_of_Acc output; Roll_orientation_of_Acc output; Z_orientation_of_Acc output; Y_value_of_Acc input; Z_value_of_Acc input
% Computing orientation of tri-axial acclerometer data from IMU 
% Author: RM van Rensburg
% Date: 26-04-2015
% Version: 1.0,tested on Matlab R2015a

function [Pitch_orientation_of_Acc,...
          Roll_orientation_of_Acc,...
          Z_orientation_of_Acc]...
          = OrientationFcn(X_value_of_Acc,Y_value_of_Acc,Z_value_of_Acc)
     
      
% Using x and y from accelerometer (g-forces), calculate x and y angles
% Data directly obtained from IMU
% Using the following formulae
% Ax = arctan{X/sqrt(Y*Y + Z*Z)}
% Ay = arctan{Y/sqrt(X*X + Z*Z)}

% Computing the X*X, Y*Y, Z*Z
X2 = power(X_value_of_Acc,2);
Y2 = power(Y_value_of_Acc,2);
Z2 = power(Z_value_of_Acc,2);

% x-axis angle
result = sqrt(Y2 + Z2);
result = X_value_of_Acc / result;
x_angle_rad = atan(result);
Pitch_orientation_of_Acc = (x_angle_rad * 180) / pi;

% y-axis angle
result = sqrt(X2 + Z2);
result = Y_value_of_Acc / result;
y_angle_rad = atan(result);
Roll_orientation_of_Acc = -(y_angle_rad * 180) / pi;

% z-axis angle
result = sqrt(Y2 + X2);
result = Z_value_of_Acc / result;
z_angle_rad = atan(result);
Z_orientation_of_Acc = (z_angle_rad * 180) / pi;

end

== matlab function kalmanAndroidAHRS/Initial Angles by Accelerometer/MATLAB Function1 ==
  data: u input; y output
function y = fcn(u)

if(isnan(u))
y=0;
else
y=u;
end

== matlab function kalmanAndroidAHRS/Subsystem1/Linear Kalman Filter Roll ==
  data: Ts input; Q_angle input; Q_bias input; R input; newAngle input; rate output; newRate input; angle_ output; bias output; P_ output; y output; K output
% Algorithm -- implimentation of Linear-Kalman filter for a 6-DOF IMU using
% a single axis for testing. A single axis consisting of both anaccelerometer
% input and gyroscope input from IMU.
% Author: RM van Rensburg
% for IMU testing purposes
% Date: 26-04-2015
% Version: 1.0,tested on Matlab R2015a

function [rate,angle_,bias,P_,y,K] = Kalmanf(Ts,...
                                             Q_angle,Q_bias,R,...
                                             newAngle,...
                                             newRate)
                      
% Process noise covariance matrix  
Q = [Q_angle 0;0 Q_bias]*Ts;
A = [1  -Ts;0  1];
C = [1 0];
bias = 0.0;

rate = newRate - bias;

persistent angle;
if isempty(angle);angle = 0;
else angle = angle + (Ts * rate); 
end
angle_= angle;
                    
persistent P;
if isempty(P);P = [0 0 ; 0 0]; 
else P = A*P*A' + Q;
end
P_=P;

S = C*P*C' + R; % Estimate error 
K = (P_*C')/S; % Kalman gain
y = newAngle - angle_; % Angle difference 
xk = angle_ + K*y;
angle_ = xk(1);
bias = xk(2);
angle = angle_;

% Update the error covariance 
I = [1 0;0 1];
P_ = (I - K*C)*P_;
% or
% Joseph form (more stable)
% P_ = (I - K*C)*P_*(I - K*C) + K*R*K';
P = P_;

return

end

== matlab function kalmanAndroidAHRS/Heading and Yaw Estimation/MATLAB Function ==
  data: a input; heading output; h input; pitch_rad input; roll_rad input
function heading  = mag2Heading(a,h,pitch_rad,roll_rad)
 a = normalize(a,'norm');
 h = normalize(h,'norm');
   
    heading_rad = atan2(h(3) * sin(roll_rad) - h(2) * cos(roll_rad), h(1) * cos(pitch_rad) + h(2) * sin(pitch_rad) * sin(roll_rad) + h(3) * sin(pitch_rad) * cos(roll_rad));
    heading = rad2deg(heading_rad);

== matlab function kalmanAndroidAHRS/Heading and Yaw Estimation/Linear Kalman Filter Heading ==
  data: Ts input; Q_angle input; Q_bias input; R input; newAngle input; rate output; newRate input; angle_ output; bias output; P_ output; y output; K output
% Algorithm -- implimentation of Linear-Kalman filter for a 6-DOF IMU using
% a single axis for testing. A single axis consisting of both anaccelerometer
% input and gyroscope input from IMU.
% Author: RM van Rensburg
% for IMU testing purposes
% Date: 26-04-2015
% Version: 1.0,tested on Matlab R2015a

function [rate,angle_,bias,P_,y,K] = Kalmanf(Ts,...
                                             Q_angle,Q_bias,R,...
                                             newAngle,...
                                             newRate)
                      
% Process noise covariance matrix  
Q = [Q_angle 0;0 Q_bias]*Ts;
A = [1  -Ts;0  1];
C = [1 0];
bias = 0.0;

rate = newRate - bias;

persistent angle;
if isempty(angle);angle = 0;
else angle = angle + (Ts * rate); 
end
 
angle_= angle;


                    
persistent P;
if isempty(P);P = [0 0 ; 0 0]; 
else P = A*P*A' + Q;
end
P_=P;

S = C*P*C' + R; % Estimate error 
K = (P_*C')/S; % Kalman gain
y = newAngle - angle_; % Angle difference 
xk = angle_ + K*y;
angle_ = xk(1);

bias = xk(2);
angle = angle_;

% Update the error covariance 
I = [1 0;0 1];
P_ = (I - K*C)*P_;
% or
% Joseph form (more stable)
% P_ = (I - K*C)*P_*(I - K*C) + K*R*K';
P = P_;


    if angle_ > 360 
        angle_ = angle_ - 360;
    elseif angle_ < 0
       angle_ =  angle_ + 360;
    end

return

end

== matlab function kalmanAndroidAHRS/Heading and Yaw Estimation/MATLAB Function3 ==
  data: u input; y output
function y = fcn(u)

if(isnan(u))
y=0;
else
y=u;
end

== matlab function kalmanAndroidAHRS/Heading and Yaw Estimation/MATLAB Function4 ==
  data: rawAngle input; angle_ output
function angle_ = constrainerHeading(rawAngle)
angle_ = rawAngle;
    if rawAngle > 360 ;
        angle_ = rawAngle - 360;
    elseif angle_ < 0;
       angle_ =  rawAngle + 360;
    end
end
